simulink model "sampleModel653"  (R2023a)
settings: Solver=VariableStepAuto  StartTime=0.0  StopTime=10.0  RelTol=1e-3
undefined symbols (not defined in the file): DiscIntNeverNeededParam, magnitude, Newton, Raphson
libraries: simulink x238, slpidlib x68
(part 8 of 11)

== system sampleModel653/cfblk160/cfblk6 ==
  cfblk1 : Inport
  cfblk8 : Inport  Port=2
  cfblk3 : Delay  SampleTime=1
  cfblk4 : DiscreteFir  SampleTime=1
  cfblk5 : DiscreteFilter  SampleTime=1
  cfblk6 : Abs  SaturateOnIntegerOverflow=off
  cfblk7 : Signum
  cfblk2 : Outport
  cfblk9 : Outport  Port=2
  cfblk10 : Outport  Port=3
  wires:
  cfblk3/1 -> cfblk9/1
  cfblk1/1 -> cfblk6/1
  cfblk8/1 -> cfblk7/1, cfblk5/1
  cfblk5/1 -> cfblk2/1
  cfblk7/1 -> cfblk10/1
  cfblk6/1 -> cfblk4/1
  cfblk4/1 -> cfblk3/1

== system sampleModel653/cfblk160/cfblk7 ==
  cfblk1 : Inport
  cfblk7 : Inport  Port=2
  cfblk3 : slpidlib/PID Controller  Controller=PID  Form=Parallel  TimeDomain=Discrete-time  UseExternalTs=off  SampleTime=1  IntegratorMethod=Forward Euler  FilterMethod=Forward Euler  ControllerParametersSource=internal  P=1  I=1  UseKiTs=off  D=0  N=100  UseFilter=on  TunerSelectOption=Transfer Function Based (PID Tuner App)  InitialConditionSource=internal  InitialConditionForIntegrator=0  InitialConditionForFilter=0  DifferentiatorICPrevScaledInput=0  ExternalReset=none  TrackingMode=off  Kt=1  LimitOutput=off  SatLimitsSource=internal  UpperSaturationLimit=inf  LowerSaturationLimit=-inf  LinearizeAsGain=off  AntiWindupMode=none  Kb=1  LimitIntegrator=off  UpperIntegratorSaturationLimit=inf  LowerIntegratorSaturationLimit=-inf  POutMin=[]  POutMax=[]  IOutMin=[]  IOutMax=[]  DOutMin=[]  DOutMax=[]  NOutMin=[]  NOutMax=[]  SumOutMin=[]  SumOutMax=[]  SaturationOutMin=[]  SaturationOutMax=[]  PParamMin=[]  PParamMax=[]  IParamMin=[]  IParamMax=[]  DParamMin=[]  DParamMax=[]  NParamMin=[]  NParamMax=[]  KbParamMin=[]  KbParamMax=[]  KtParamMin=[]  KtParamMax=[]  KbOutMin=[]  KbOutMax=[]  KtOutMin=[]  KtOutMax=[]  IntegratorOutMin=[]  IntegratorOutMax=[]  FilterOutMin=[]  FilterOutMax=[]  SumI1OutMin=[]  SumI1OutMax=[]  SumI2OutMin=[]  SumI2OutMax=[]  SumI3OutMin=[]  SumI3OutMax=[]  SumI4OutMin=[]  SumI4OutMax=[]  SumDOutMin=[]  SumDOutMax=[]  DifferentiatorOutMin=[]  DifferentiatorOutMax=[]  FilterDiffOutCoefMin=[]  FilterDiffOutCoefMax=[]  ReciprocalOutMin=[]  ReciprocalOutMax=[]  SumDenOutMin=[]  SumDenOutMax=[]  SumNumOutMin=[]  SumNumOutMax=[]  DivideOutMin=[]  DivideOutMax=[]  UdiffTsProdOutMin=[]  UdiffTsProdOutMax=[]  NTsProdOutMin=[]  NTsProdOutMax=[]  UintegralTsProdOutMin=[]  UintegralTsProdOutMax=[]  UngainTsProdOutMin=[]  UngainTsProdOutMax=[]  ClampingZeroOutDataTypeStr=Inherit: Inherit via back propagation  ClampingZeroOutMin=[]  ClampingZeroOutMax=[]  FilterDenConstantOutDataTypeStr=Inherit: Inherit via back propagation  FilterDenConstantOutMin=[]  FilterDenConstantOutMax=[]  PCopyOutDataTypeStr=Inherit: Inherit via back propagation  PCopyOutMin=[]  PCopyOutMax=[]  NCopyOutDataTypeStr=Inherit: Inherit via back propagation  NCopyOutMin=[]  NCopyOutMax=[]  IntegratorContinuousStateAttributes=''  IntegratorStateMustResolveToSignalObject=off  IntegratorRTWStateStorageClass=Auto  FilterContinuousStateAttributes=''  FilterStateMustResolveToSignalObject=off  FilterRTWStateStorageClass=Auto  ParallelPVariant=InternalParameters  IdealPVariant=Disabled  IVariant=InternalParameters  DVariant=InternalParameters  IntegratorVariant=Discrete  SatVariant=Disabled  AWVariant=Passthrough  PCopyVariant=Disabled  TRVariant=Disabled  FdbkBlocksVariant=Forward  IdealPFdbkVariant=Disabled  SatFdbkVariant=Disabled  DerivativeFilterVariant=ForwardEulerFilter  NVariant=InternalParameters  NCopyVariant=Disabled  FilterICVariant=InternalICsFilter  IntegratorICVariant=InternalICs  ExternalResetVariant=Disabled  TRSumVariant=Passthrough  SumFdbkVariant=Disabled  SumVariant=Sum_PID  TsampFilterVariant=InternalTs  TsampNgainVariant=Passthrough  TsampIntegralVariant=Disabled_SignalSpec  ExternalSaturationOutDataTypeStr=Inherit: Same as second input
      settings: LibrarySourceBlock=simulink/Discrete/Discrete PID Controller
  cfblk4 : Sum  Inputs=|++
  cfblk5 : Polyval  Coefs=[ +2.081618890e-019, -1.441693666e-014, +4.719686976e-010, -8.536869453e-006, +1.621573104e-001, -8.087801117e+001 ]
  cfblk6 : Constant  Value=[-549633033.894766]  SampleTime=1
  cfblk2 : Outport
  wires:
  cfblk6/1 -> cfblk2/1
  cfblk7/1 -> cfblk3/1
  cfblk3/1 -> cfblk4/1
  cfblk1/1 -> cfblk4/2
  cfblk4/1 -> cfblk5/1

== system sampleModel653/cfblk161/cfblk13 ==
  cfblk1 : Inport
  cfblk13 : Inport  Port=2
  cfblk10 : Product
  cfblk11 : Constant  Value=[950367817.436596]  SampleTime=1
  cfblk12 : Constant  Value=[-836391739.954289]  SampleTime=1
  cfblk16 : Delay  SampleTime=1
  cfblk17 : Delay  SampleTime=1
  cfblk3 : PropagationDelay  SampleTime=1
  cfblk4 : simulink/Discrete/Transfer Fcn First Order  PoleZ=0.95  ICPrevOutput=0.0  DoSatur=off
  cfblk5 : simulink/Discrete/Tapped Delay  vinit=0.0  samptime=-1  NumDelays=1  DelayOrder=Oldest  includeCurrent=off
  cfblk6 : PropagationDelay  SampleTime=1
  cfblk7 : Sum  Inputs=+-
  cfblk8 : ComplexToMagnitudeAngle
  cfblk9 : Sqrt
  cfblk2 : Outport
  cfblk14 : Outport  Port=2
  cfblk15 : Outport  Port=3
  wires:
  cfblk3/1 -> cfblk4/1
  cfblk12/1 -> cfblk9/1
  cfblk1/1 -> cfblk6/1
  cfblk7/1 -> cfblk8/1
  cfblk13/1 -> cfblk15/1
  cfblk5/1 -> cfblk14/1, cfblk10/2
  cfblk4/1 -> cfblk6/2
  cfblk6/1 -> cfblk2/1
  cfblk8/2 -> cfblk10/1
  cfblk9/1 -> cfblk7/2, cfblk3/2
  cfblk11/1 -> cfblk3/1
  cfblk10/1 -> cfblk16/1
  cfblk16/1 -> cfblk5/1
  cfblk8/1 -> cfblk17/1
  cfblk17/1 -> cfblk7/1

== system sampleModel653/cfblk161/cfblk14 ==
  cfblk1 : Inport
  cfblk6 : Inport  Port=2
  cfblk3 : MinMax  Function=max  Inputs=3
  cfblk4 : Constant  Value=[-385450428.732004]  SampleTime=1
  cfblk5 : Constant  Value=[-397891502.363819]  SampleTime=1
  cfblk2 : Outport
  cfblk7 : Outport  Port=2
  cfblk8 : Outport  Port=3
  wires:
  cfblk5/1 -> cfblk7/1
  cfblk6/1 -> cfblk8/1, cfblk3/2
  cfblk1/1 -> cfblk2/1
  cfblk4/1 -> cfblk3/1, cfblk3/3

== system sampleModel653/cfblk162/cfblk10 ==
  cfblk1 : Inport
  cfblk6 : Inport  Port=2
  cfblk3 : DiscreteIntegrator  ICPrevOutput=DiscIntNeverNeededParam  ICPrevScaledInput=DiscIntNeverNeededParam
  cfblk4 : Sqrt  Operator=rSqrt  AlgorithmType=Newton-Raphson
  cfblk5 : Sum  Inputs=--
  cfblk2 : Outport
  cfblk7 : Outport  Port=2
  wires:
  cfblk1/1 -> cfblk4/1
  cfblk6/1 -> cfblk2/1, cfblk5/2
  cfblk3/1 -> cfblk7/1, cfblk5/1
  cfblk4/1 -> cfblk3/1

== system sampleModel653/cfblk162/cfblk11 ==
  cfblk1 : Inport
  cfblk14 : Inport  Port=2
  cfblk15 : Inport  Port=3
  cfblk16 : Inport  Port=4
  cfblk10 : Gain  Gain=[646766458.075510]
  cfblk11 : Constant  Value=[-624023355.603475]  SampleTime=1
  cfblk12 : Constant  Value=[-240685083.837348]  SampleTime=1
  cfblk13 : Constant  Value=[301386795.855852]  SampleTime=1
  cfblk3 : DiscreteIntegrator  ICPrevOutput=DiscIntNeverNeededParam  ICPrevScaledInput=DiscIntNeverNeededParam
  cfblk4 : UnaryMinus
  cfblk5 : Trigonometry
  cfblk6 : Math  Operator=rem
  cfblk7 : UnaryMinus
  cfblk8 : Signum
  cfblk9 : simulink/Math Operations/Slider Gain  gain=1  low=0  high=2
  cfblk2 : Outport
  wires:
  cfblk15/1 -> cfblk6/1
  cfblk12/1 -> cfblk6/2
  cfblk16/1 -> cfblk2/1
  cfblk4/1 -> cfblk9/1
  cfblk14/1 -> cfblk7/1
  cfblk10/1 -> cfblk3/1
  cfblk11/1 -> cfblk4/1
  cfblk13/1 -> cfblk10/1
  cfblk6/1 -> cfblk8/1
  cfblk9/1 -> cfblk5/1

== system sampleModel653/cfblk162/cfblk7 ==
  cfblk1 : Inport
  cfblk13 : Inport  Port=2
  cfblk14 : Inport  Port=3
  cfblk10 : PermuteDimensions
  cfblk11 : Constant  Value=[11170143.397461]  SampleTime=1
  cfblk12 : Constant  Value=[-707565245.150474]  SampleTime=1
  cfblk17 : Delay  SampleTime=1
  cfblk3 : DiscreteTransferFcn  SampleTime=1
  cfblk4 : ComplexToMagnitudeAngle
  cfblk5 : DotProduct  OutDataTypeStr=Inherit: Inherit via internal rule
  cfblk6 : Bias  Bias=[-243802448.870084]  SaturateOnIntegerOverflow=off
  cfblk7 : Bias  Bias=[722005986.652119]  SaturateOnIntegerOverflow=off
  cfblk8 : Sum  Inputs=+-
  cfblk9 : PermuteDimensions
  cfblk2 : Outport
  cfblk15 : Outport  Port=2
  cfblk16 : Outport  Port=3
  wires:
  cfblk3/1 -> cfblk10/1
  cfblk1/1 -> cfblk3/1
  cfblk10/1 -> cfblk5/2
  cfblk13/1 -> cfblk6/1
  cfblk7/1 -> cfblk15/1
  cfblk14/1 -> cfblk2/1
  cfblk4/1 -> cfblk9/1
  cfblk11/1 -> cfblk16/1
  cfblk6/1 -> cfblk4/1
  cfblk12/1 -> cfblk7/1
  cfblk4/2 -> cfblk8/1
  cfblk5/1 -> cfblk8/2
  cfblk8/1 -> cfblk17/1
  cfblk17/1 -> cfblk5/1

== system sampleModel653/cfblk162/cfblk8 ==
  cfblk1 : Inport
  cfblk7 : Inport  Port=2
  cfblk8 : Inport  Port=3
  cfblk3 : DiscreteFilter  SampleTime=1
  cfblk4 : PermuteDimensions
  cfblk5 : Trigonometry
  cfblk6 : Constant  Value=[643614640.202509]  SampleTime=1
  cfblk2 : Outport
  cfblk9 : Outport  Port=2
  cfblk10 : Outport  Port=3
  wires:
  cfblk8/1 -> cfblk3/1
  cfblk3/1 -> cfblk2/1
  cfblk6/1 -> cfblk5/1
  cfblk7/1 -> cfblk9/1
  cfblk1/1 -> cfblk4/1
  cfblk5/1 -> cfblk10/1

== system sampleModel653/cfblk162/cfblk9 ==
  cfblk1 : Inport
  cfblk14 : Inport  Port=2
  cfblk15 : Inport  Port=3
  cfblk10 : Sum  Inputs=|++
  cfblk11 : Bias  Bias=[360480806.140065]  SaturateOnIntegerOverflow=off
  cfblk12 : Bias  Bias=[-571993292.003574]  SaturateOnIntegerOverflow=off
  cfblk13 : Constant  Value=[994996432.571754]  SampleTime=1
  cfblk18 : Delay  SampleTime=1
  cfblk3 : DiscreteStateSpace
  cfblk4 : DiscreteTransferFcn  SampleTime=1
  cfblk5 : Sum  Inputs=+-
  cfblk6 : PermuteDimensions
  cfblk7 : Product  Inputs=**
  cfblk8 : Polyval  Coefs=[ +2.081618890e-019, -1.441693666e-014, +4.719686976e-010, -8.536869453e-006, +1.621573104e-001, -8.087801117e+001 ]
  cfblk9 : simulink/Math Operations/Slider Gain  gain=1  low=0  high=2
  cfblk2 : Outport
  cfblk16 : Outport  Port=2
  cfblk17 : Outport  Port=3
  wires:
  cfblk7/1 -> cfblk9/1
  cfblk13/1 -> cfblk4/1
  cfblk15/1 -> cfblk16/1, cfblk5/2
  cfblk5/1 -> cfblk11/1
  cfblk14/1 -> cfblk17/1
  cfblk3/1 -> cfblk12/1, cfblk10/2
  cfblk11/1 -> cfblk6/1
  cfblk6/1 -> cfblk8/1
  cfblk8/1 -> cfblk7/2
  cfblk4/1 -> cfblk3/1
  cfblk9/1 -> cfblk10/1
  cfblk12/1 -> cfblk2/1
  cfblk1/1 -> cfblk5/1
  cfblk10/1 -> cfblk18/1
  cfblk18/1 -> cfblk7/1

== system sampleModel653/cfblk164/cfblk6 ==
  cfblk1 : Inport
  cfblk12 : Inport  Port=2
  cfblk13 : Inport  Port=3
  cfblk14 : Inport  Port=4
  cfblk15 : Inport  Port=5
  cfblk10 : Sum  Inputs=|++
  cfblk11 : Constant  Value=[-495831747.565326]  SampleTime=1
  cfblk16 : Delay  SampleTime=1
  cfblk3 : DiscreteZeroPole  Poles=[0 0.5]  Gain=1
  cfblk4 : Polyval  Coefs=[ +2.081618890e-019, -1.441693666e-014, +4.719686976e-010, -8.536869453e-006, +1.621573104e-001, -8.087801117e+001 ]
  cfblk5 : Product  Inputs=*
  cfblk6 : Polyval  Coefs=[ +2.081618890e-019, -1.441693666e-014, +4.719686976e-010, -8.536869453e-006, +1.621573104e-001, -8.087801117e+001 ]
  cfblk7 : MinMax
  cfblk8 : Sum  Inputs=+-
  cfblk9 : Gain  Gain=[160082621.041348]
  cfblk2 : Outport
  wires:
  cfblk12/1 -> cfblk6/1
  cfblk13/1 -> cfblk4/1
  cfblk4/1 -> cfblk2/1
  cfblk11/1 -> cfblk7/1
  cfblk15/1 -> cfblk9/1
  cfblk6/1 -> cfblk5/1
  cfblk3/1 -> cfblk8/1
  cfblk10/1 -> cfblk8/2
  cfblk9/1 -> cfblk10/1
  cfblk7/1 -> cfblk10/2
  cfblk8/1 -> cfblk16/1
  cfblk16/1 -> cfblk3/1

== system sampleModel653/cfblk165/cfblk7 ==
  cfblk1 : Inport
  cfblk3 : DiscreteTransferFcn  SampleTime=1
  cfblk4 : Gain  Gain=[-702568927.558802]
  cfblk5 : Product  Inputs=*
  cfblk8 : Delay  SampleTime=1
  cfblk2 : Outport
  cfblk6 : Outport  Port=2
  cfblk7 : Outport  Port=3
  wires:
  cfblk1/1 -> cfblk2/1, cfblk4/1
  cfblk4/1 -> cfblk7/1
  cfblk3/1 -> cfblk6/1, cfblk5/1
  cfblk5/1 -> cfblk8/1
  cfblk8/1 -> cfblk3/1

== system sampleModel653/cfblk166/cfblk7 ==
  cfblk1 : Inport
  cfblk10 : Inport  Port=2
  cfblk11 : Inport  Port=3
  cfblk12 : Inport  Port=4
  cfblk13 : Inport  Port=5
  cfblk14 : Inport  Port=6
  cfblk15 : Inport  Port=7
  cfblk3 : PropagationDelay  SampleTime=1
  cfblk4 : DiscreteFilter  SampleTime=1
  cfblk5 : DiscreteFilter  SampleTime=1
  cfblk6 : UnitDelay  HasFrameUpgradeWarning=on
  cfblk7 : PermuteDimensions
  cfblk8 : Bias  Bias=[88992789.129511]  SaturateOnIntegerOverflow=off
  cfblk9 : Constant  Value=[-39645168.443005]  SampleTime=1
  cfblk2 : Outport
  wires:
  cfblk12/1 -> cfblk8/1
  cfblk1/1 -> cfblk5/1
  cfblk10/1 -> cfblk6/1
  cfblk14/1 -> cfblk4/1
  cfblk11/1 -> cfblk3/1
  cfblk9/1 -> cfblk3/2
  cfblk4/1 -> cfblk7/1
  cfblk6/1 -> cfblk2/1

== system sampleModel653/cfblk167/cfblk10 ==
  cfblk1 : Inport
  cfblk9 : Inport  Port=2
  cfblk11 : Delay  SampleTime=1
  cfblk12 : Delay  SampleTime=1
  cfblk3 : PropagationDelay  SampleTime=1
  cfblk4 : PropagationDelay  SampleTime=1
  cfblk5 : DiscreteZeroPole  Poles=[0 0.5]  Gain=1
  cfblk6 : Product  Inputs=**
  cfblk7 : MinMax  Inputs=3
  cfblk8 : Sum  Inputs=|++
  cfblk2 : Outport
  cfblk10 : Outport  Port=2
  wires:
  cfblk9/1 -> cfblk5/1
  cfblk5/1 -> cfblk10/1
  cfblk3/1 -> cfblk4/1, cfblk8/1
  cfblk8/1 -> cfblk6/2, cfblk12/1
  cfblk4/1 -> cfblk6/1
  cfblk1/1 -> cfblk7/2, cfblk7/3
  cfblk7/1 -> cfblk2/1, cfblk3/1, cfblk3/2, cfblk8/2
  cfblk6/1 -> cfblk11/1
  cfblk11/1 -> cfblk4/2
  cfblk12/1 -> cfblk7/1

== system sampleModel653/cfblk167/cfblk11 ==
  cfblk1 : Inport
  cfblk14 : Inport  Port=2
  cfblk15 : Inport  Port=3
  cfblk10 : DotProduct  OutDataTypeStr=Inherit: Inherit via internal rule
  cfblk11 : Sqrt  Operator=rSqrt  AlgorithmType=Newton-Raphson
  cfblk12 : Sum  Inputs=|++
  cfblk13 : Product  Inputs=*
  cfblk{17..20} (4 alike) : Delay  SampleTime=1
  cfblk3 : DiscreteFilter  SampleTime=1
  cfblk4 : PropagationDelay  SampleTime=1
  cfblk5 : PropagationDelay  SampleTime=1
  cfblk6 : Signum
  cfblk7 : MinMax  Function=max  Inputs=2
  cfblk8 : Sum  Inputs=|++
  cfblk9 : DotProduct  OutDataTypeStr=Inherit: Inherit via internal rule
  cfblk2 : Outport
  cfblk16 : Outport  Port=2
  wires:
  cfblk9/1 -> cfblk8/1, cfblk7/1
  cfblk13/1 -> cfblk5/1, cfblk8/2, cfblk2/1
  cfblk8/1 -> cfblk7/2, cfblk18/1
  cfblk6/1 -> cfblk4/2
  cfblk4/1 -> cfblk10/1
  cfblk14/1 -> cfblk13/1
  cfblk1/1 -> cfblk3/1
  cfblk10/1 -> cfblk12/2, cfblk9/2
  cfblk3/1 -> cfblk16/1
  cfblk5/1 -> cfblk11/1
  cfblk12/1 -> cfblk9/1, cfblk17/1
  cfblk15/1 -> cfblk6/1
  cfblk17/1 -> cfblk10/2
  cfblk18/1 -> cfblk4/1
  cfblk7/1 -> cfblk19/1
  cfblk19/1 -> cfblk12/1
  cfblk11/1 -> cfblk20/1
  cfblk20/1 -> cfblk5/2

== system sampleModel653/cfblk167/cfblk12 ==
  cfblk1 : Inport
  cfblk10 : Inport  Port=2
  cfblk11 : Inport  Port=3
  cfblk12 : Delay  SampleTime=1
  cfblk3 : Product
  cfblk4 : simulink/Math Operations/MinMax Running Resettable  Function=min  vinit=0.0
  cfblk5 : Assignment  DiagnosticForDimensions=Warning  IndexOptions=Index vector (dialog)  Indices=1  OutputSizes=1
  cfblk6 : Math  Operator=hermitian
  cfblk7 : MinMax  Inputs=2
  cfblk8 : Constant  Value=[598638791.234022]  SampleTime=1
  cfblk9 : Constant  Value=[471752082.064048]  SampleTime=1
  cfblk2 : Outport
  wires:
  cfblk8/1 -> cfblk7/1
  cfblk9/1 -> cfblk6/1
  cfblk1/1 -> cfblk7/2
  cfblk3/1 -> cfblk5/1
  cfblk6/1 -> cfblk3/1
  cfblk10/1 -> cfblk5/2
  cfblk11/1 -> cfblk4/1
  cfblk5/1 -> cfblk4/2
  cfblk7/1 -> cfblk2/1
  cfblk4/1 -> cfblk12/1
  cfblk12/1 -> cfblk3/2

== system sampleModel653/cfblk167/cfblk13 ==
  cfblk1 : Inport
  cfblk15 : Inport  Port=2
  cfblk16 : Inport  Port=3
  cfblk10 : Trigonometry
  cfblk11 : MinMax  Function=max  Inputs=2
  cfblk12 : Assignment  DiagnosticForDimensions=Warning  IndexOptions=Index vector (dialog)  Indices=1  OutputSizes=1
  cfblk13 : Constant  Value=[580497405.905219]  SampleTime=1
  cfblk14 : Constant  Value=[-757720306.002820]  SampleTime=1
  cfblk3 : UnitDelay  HasFrameUpgradeWarning=on
  cfblk4 : Gain  Gain=[619591310.488416]
  cfblk5 : DotProduct  OutDataTypeStr=Inherit: Inherit via internal rule
  cfblk6 : Math  Operator=10^u
  cfblk7 : PermuteDimensions
  cfblk8 : Product  Inputs=*
  cfblk9 : Sqrt  Operator=rSqrt  AlgorithmType=Newton-Raphson
  cfblk2 : Outport
  cfblk17 : Outport  Port=2
  wires:
  cfblk6/1 -> cfblk8/1
  cfblk14/1 -> cfblk12/1
  cfblk4/1 -> cfblk10/1
  cfblk10/1 -> cfblk7/1
  cfblk9/1 -> cfblk12/2
  cfblk15/1 -> cfblk9/1
  cfblk1/1 -> cfblk5/1
  cfblk11/1 -> cfblk6/1
  cfblk5/1 -> cfblk4/1
  cfblk8/1 -> cfblk17/1
  cfblk7/1 -> cfblk3/1
  cfblk13/1 -> cfblk2/1
  cfblk3/1 -> cfblk11/1
  cfblk16/1 -> cfblk11/2
  cfblk12/1 -> cfblk5/2

== system sampleModel653/cfblk167/cfblk18 ==
  cfblk1 : Inport
  cfblk10 : Inport  Port=2
  cfblk11 : Inport  Port=3
  cfblk12 : Inport  Port=4
  Action Port : ActionPort  ActionPortLabel=if(u1 >= 0)
  cfblk3 : simulink/Discrete/Transfer Fcn First Order  PoleZ=0.95  ICPrevOutput=0.0  DoSatur=off
  cfblk4 : DiscreteFir
  cfblk5 : Delay  ShowEnablePort=on
      settings: InputPortMap=u0,e6
  cfblk6 : DiscreteZeroPole  Poles=[0 0.5]  Gain=1  SampleTime=-1
  cfblk7 : Polyval  Coefs=[ +2.081618890e-019, -1.441693666e-014, +4.719686976e-010, -8.536869453e-006, +1.621573104e-001, -8.087801117e+001 ]
  cfblk8 : Constant  Value=[815668544.395762]  SampleTime=1
  cfblk9 : Constant  Value=[749946664.486062]  SampleTime=1
  cfblk2 : Outport
  cfblk13 : Outport  Port=2
  wires:
  cfblk10/1 -> cfblk5/1
  cfblk4/1 -> cfblk13/1
  cfblk12/1 -> cfblk5/2
  cfblk8/1 -> cfblk6/1
  cfblk11/1 -> cfblk7/1
  cfblk5/1 -> cfblk4/1
  cfblk3/1 -> cfblk2/1
  cfblk6/1 -> cfblk3/1

== system sampleModel653/cfblk167/cfblk19 ==
  cfblk1 : Inport
  cfblk13 : Inport  Port=2
  cfblk14 : Inport  Port=3
  cfblk15 : Inport  Port=4
  Action Port : ActionPort  ActionPortLabel=else
  cfblk10 : Product
  cfblk11 : Constant  Value=[365730879.526834]  SampleTime=1
  cfblk12 : Constant  Value=[357784295.505413]  SampleTime=1
  cfblk18 : Delay
  cfblk3 : PropagationDelay  SampleTime=-1
  cfblk4 : slpidlib/PID Controller  Controller=PID  Form=Parallel  TimeDomain=Discrete-time  UseExternalTs=off  SampleTime=-1  IntegratorMethod=Forward Euler  FilterMethod=Forward Euler  ControllerParametersSource=internal  P=1  I=1  UseKiTs=off  D=0  N=100  UseFilter=on  TunerSelectOption=Transfer Function Based (PID Tuner App)  InitialConditionSource=internal  InitialConditionForIntegrator=0  InitialConditionForFilter=0  DifferentiatorICPrevScaledInput=0  ExternalReset=none  TrackingMode=off  Kt=1  LimitOutput=off  SatLimitsSource=internal  UpperSaturationLimit=inf  LowerSaturationLimit=-inf  LinearizeAsGain=off  AntiWindupMode=none  Kb=1  LimitIntegrator=off  UpperIntegratorSaturationLimit=inf  LowerIntegratorSaturationLimit=-inf  POutMin=[]  POutMax=[]  IOutMin=[]  IOutMax=[]  DOutMin=[]  DOutMax=[]  NOutMin=[]  NOutMax=[]  SumOutMin=[]  SumOutMax=[]  SaturationOutMin=[]  SaturationOutMax=[]  PParamMin=[]  PParamMax=[]  IParamMin=[]  IParamMax=[]  DParamMin=[]  DParamMax=[]  NParamMin=[]  NParamMax=[]  KbParamMin=[]  KbParamMax=[]  KtParamMin=[]  KtParamMax=[]  KbOutMin=[]  KbOutMax=[]  KtOutMin=[]  KtOutMax=[]  IntegratorOutMin=[]  IntegratorOutMax=[]  FilterOutMin=[]  FilterOutMax=[]  SumI1OutMin=[]  SumI1OutMax=[]  SumI2OutMin=[]  SumI2OutMax=[]  SumI3OutMin=[]  SumI3OutMax=[]  SumI4OutMin=[]  SumI4OutMax=[]  SumDOutMin=[]  SumDOutMax=[]  DifferentiatorOutMin=[]  DifferentiatorOutMax=[]  FilterDiffOutCoefMin=[]  FilterDiffOutCoefMax=[]  ReciprocalOutMin=[]  ReciprocalOutMax=[]  SumDenOutMin=[]  SumDenOutMax=[]  SumNumOutMin=[]  SumNumOutMax=[]  DivideOutMin=[]  DivideOutMax=[]  UdiffTsProdOutMin=[]  UdiffTsProdOutMax=[]  NTsProdOutMin=[]  NTsProdOutMax=[]  UintegralTsProdOutMin=[]  UintegralTsProdOutMax=[]  UngainTsProdOutMin=[]  UngainTsProdOutMax=[]  ClampingZeroOutDataTypeStr=Inherit: Inherit via back propagation  ClampingZeroOutMin=[]  ClampingZeroOutMax=[]  FilterDenConstantOutDataTypeStr=Inherit: Inherit via back propagation  FilterDenConstantOutMin=[]  FilterDenConstantOutMax=[]  PCopyOutDataTypeStr=Inherit: Inherit via back propagation  PCopyOutMin=[]  PCopyOutMax=[]  NCopyOutDataTypeStr=Inherit: Inherit via back propagation  NCopyOutMin=[]  NCopyOutMax=[]  IntegratorContinuousStateAttributes=''  IntegratorStateMustResolveToSignalObject=off  IntegratorRTWStateStorageClass=Auto  FilterContinuousStateAttributes=''  FilterStateMustResolveToSignalObject=off  FilterRTWStateStorageClass=Auto  ParallelPVariant=InternalParameters  IdealPVariant=Disabled  IVariant=InternalParameters  DVariant=InternalParameters  IntegratorVariant=Discrete  SatVariant=Disabled  AWVariant=Passthrough  PCopyVariant=Disabled  TRVariant=Disabled  FdbkBlocksVariant=Forward  IdealPFdbkVariant=Disabled  SatFdbkVariant=Disabled  DerivativeFilterVariant=ForwardEulerFilter  NVariant=InternalParameters  NCopyVariant=Disabled  FilterICVariant=InternalICsFilter  IntegratorICVariant=InternalICs  ExternalResetVariant=Disabled  TRSumVariant=Passthrough  SumFdbkVariant=Disabled  SumVariant=Sum_PID  TsampFilterVariant=InternalTs  TsampNgainVariant=Passthrough  TsampIntegralVariant=Disabled_SignalSpec  ExternalSaturationOutDataTypeStr=Inherit: Same as second input
      settings: LibrarySourceBlock=simulink/Discrete/Discrete PID Controller
  cfblk5 : Delay
  cfblk6 : DiscreteStateSpace  SampleTime=-1
  cfblk7 : UnitDelay  SampleTime=-1  HasFrameUpgradeWarning=on
  cfblk8 : Signum
  cfblk9 : Sum  Inputs=+
  cfblk2 : Outport
  cfblk16 : Outport  Port=2
  cfblk17 : Outport  Port=3
  wires:
  cfblk9/1 -> cfblk10/1
  cfblk12/1 -> cfblk5/1
  cfblk5/1 -> cfblk10/2
  cfblk13/1 -> cfblk4/1
  cfblk11/1 -> cfblk17/1
  cfblk1/1 -> cfblk16/1
  cfblk14/1 -> cfblk7/1
  cfblk6/1 -> cfblk2/1
  cfblk7/1 -> cfblk6/1
  cfblk8/1 -> cfblk3/1
  cfblk3/1 -> cfblk9/1
  cfblk15/1 -> cfblk8/1
  cfblk10/1 -> cfblk18/1
  cfblk18/1 -> cfblk3/2

== system sampleModel653/cfblk167/cfblk8 ==
  cfblk1 : Inport
  cfblk3 : DiscreteFir  SampleTime=1
  cfblk4 : simulink/Discrete/Tapped Delay  vinit=0.0  samptime=-1  NumDelays=1  DelayOrder=Oldest  includeCurrent=off
  cfblk5 : Sqrt
  cfblk6 : Rounding
  cfblk9 : Delay  SampleTime=1
  cfblk2 : Outport
  cfblk7 : Outport  Port=2
  cfblk8 : Outport  Port=3
  wires:
  cfblk6/1 -> cfblk5/1, cfblk9/1
  cfblk3/1 -> cfblk6/1
  cfblk5/1 -> cfblk2/1
  cfblk1/1 -> cfblk4/1
  cfblk4/1 -> cfblk8/1, cfblk7/1
  cfblk9/1 -> cfblk3/1

== system sampleModel653/cfblk167/cfblk9 ==
  cfblk1 : Inport
  cfblk11 : Inport  Port=2
  cfblk12 : Inport  Port=3
  cfblk13 : Inport  Port=4
  cfblk14 : Inport  Port=5
  cfblk10 : Constant  Value=[484188899.570974]  SampleTime=1
  cfblk3 : Sin  TimeSource=Use external signal  SampleTime=0
  cfblk4 : Squeeze
  cfblk5 : Squeeze
  cfblk6 : Sum  Inputs=|++
  cfblk7 : Polyval  Coefs=[ +2.081618890e-019, -1.441693666e-014, +4.719686976e-010, -8.536869453e-006, +1.621573104e-001, -8.087801117e+001 ]
  cfblk8 : Sqrt  Operator=rSqrt  AlgorithmType=Newton-Raphson
  cfblk9 : Constant  Value=[327374608.869159]  SampleTime=1
  cfblk2 : Outport
  cfblk15 : Outport  Port=2
  wires:
  cfblk9/1 -> cfblk2/1
  cfblk4/1 -> cfblk8/1
  cfblk5/1 -> cfblk4/1
  cfblk10/1 -> cfblk6/1
  cfblk7/1 -> cfblk15/1
  cfblk12/1 -> cfblk3/1
  cfblk11/1 -> cfblk5/1
  cfblk6/1 -> cfblk7/1
  cfblk3/1 -> cfblk6/2

== system sampleModel653/cfblk168/cfblk7 ==
  cfblk1 : Inport
  cfblk10 : Constant  Value=[701061649.043973]  SampleTime=1
  cfblk12 : Delay  SampleTime=1
  cfblk13 : Delay  SampleTime=1
  cfblk3 : slpidlib/PID Controller  Controller=PID  Form=Parallel  TimeDomain=Discrete-time  UseExternalTs=off  SampleTime=1  IntegratorMethod=Forward Euler  FilterMethod=Forward Euler  ControllerParametersSource=internal  P=1  I=1  UseKiTs=off  D=0  N=100  UseFilter=on  TunerSelectOption=Transfer Function Based (PID Tuner App)  InitialConditionSource=internal  InitialConditionForIntegrator=0  InitialConditionForFilter=0  DifferentiatorICPrevScaledInput=0  ExternalReset=none  TrackingMode=off  Kt=1  LimitOutput=off  SatLimitsSource=internal  UpperSaturationLimit=inf  LowerSaturationLimit=-inf  LinearizeAsGain=off  AntiWindupMode=none  Kb=1  LimitIntegrator=off  UpperIntegratorSaturationLimit=inf  LowerIntegratorSaturationLimit=-inf  POutMin=[]  POutMax=[]  IOutMin=[]  IOutMax=[]  DOutMin=[]  DOutMax=[]  NOutMin=[]  NOutMax=[]  SumOutMin=[]  SumOutMax=[]  SaturationOutMin=[]  SaturationOutMax=[]  PParamMin=[]  PParamMax=[]  IParamMin=[]  IParamMax=[]  DParamMin=[]  DParamMax=[]  NParamMin=[]  NParamMax=[]  KbParamMin=[]  KbParamMax=[]  KtParamMin=[]  KtParamMax=[]  KbOutMin=[]  KbOutMax=[]  KtOutMin=[]  KtOutMax=[]  IntegratorOutMin=[]  IntegratorOutMax=[]  FilterOutMin=[]  FilterOutMax=[]  SumI1OutMin=[]  SumI1OutMax=[]  SumI2OutMin=[]  SumI2OutMax=[]  SumI3OutMin=[]  SumI3OutMax=[]  SumI4OutMin=[]  SumI4OutMax=[]  SumDOutMin=[]  SumDOutMax=[]  DifferentiatorOutMin=[]  DifferentiatorOutMax=[]  FilterDiffOutCoefMin=[]  FilterDiffOutCoefMax=[]  ReciprocalOutMin=[]  ReciprocalOutMax=[]  SumDenOutMin=[]  SumDenOutMax=[]  SumNumOutMin=[]  SumNumOutMax=[]  DivideOutMin=[]  DivideOutMax=[]  UdiffTsProdOutMin=[]  UdiffTsProdOutMax=[]  NTsProdOutMin=[]  NTsProdOutMax=[]  UintegralTsProdOutMin=[]  UintegralTsProdOutMax=[]  UngainTsProdOutMin=[]  UngainTsProdOutMax=[]  ClampingZeroOutDataTypeStr=Inherit: Inherit via back propagation  ClampingZeroOutMin=[]  ClampingZeroOutMax=[]  FilterDenConstantOutDataTypeStr=Inherit: Inherit via back propagation  FilterDenConstantOutMin=[]  FilterDenConstantOutMax=[]  PCopyOutDataTypeStr=Inherit: Inherit via back propagation  PCopyOutMin=[]  PCopyOutMax=[]  NCopyOutDataTypeStr=Inherit: Inherit via back propagation  NCopyOutMin=[]  NCopyOutMax=[]  IntegratorContinuousStateAttributes=''  IntegratorStateMustResolveToSignalObject=off  IntegratorRTWStateStorageClass=Auto  FilterContinuousStateAttributes=''  FilterStateMustResolveToSignalObject=off  FilterRTWStateStorageClass=Auto  ParallelPVariant=InternalParameters  IdealPVariant=Disabled  IVariant=InternalParameters  DVariant=InternalParameters  IntegratorVariant=Discrete  SatVariant=Disabled  AWVariant=Passthrough  PCopyVariant=Disabled  TRVariant=Disabled  FdbkBlocksVariant=Forward  IdealPFdbkVariant=Disabled  SatFdbkVariant=Disabled  DerivativeFilterVariant=ForwardEulerFilter  NVariant=InternalParameters  NCopyVariant=Disabled  FilterICVariant=InternalICsFilter  IntegratorICVariant=InternalICs  ExternalResetVariant=Disabled  TRSumVariant=Passthrough  SumFdbkVariant=Disabled  SumVariant=Sum_PID  TsampFilterVariant=InternalTs  TsampNgainVariant=Passthrough  TsampIntegralVariant=Disabled_SignalSpec  ExternalSaturationOutDataTypeStr=Inherit: Same as second input
      settings: LibrarySourceBlock=simulink/Discrete/Discrete PID Controller
  cfblk4 : Delay  DelayLengthSource=Input port  SampleTime=1
      settings: InputPortMap=u0,p1
  cfblk5 : DiscreteFir  SampleTime=1
  cfblk6 : Assignment  DiagnosticForDimensions=Warning  IndexOptions=Index vector (dialog)  Indices=1  OutputSizes=1
  cfblk7 : UnaryMinus
  cfblk8 : Reshape
  cfblk9 : Rounding
  cfblk2 : Outport
  cfblk11 : Outport  Port=2
  wires:
  cfblk4/1 -> cfblk6/1
  cfblk3/1 -> cfblk5/1
  cfblk1/1 -> cfblk6/2
  cfblk7/1 -> cfblk9/1
  cfblk6/1 -> cfblk2/1
  cfblk9/1 -> cfblk4/1, cfblk8/1
  cfblk8/1 -> cfblk11/1, cfblk13/1
  cfblk10/1 -> cfblk4/2
  cfblk5/1 -> cfblk12/1
  cfblk12/1 -> cfblk3/1
  cfblk13/1 -> cfblk7/1

== system sampleModel653/cfblk168/cfblk8 ==
  cfblk1 : Inport
  cfblk10 : Inport  Port=2
  cfblk12 : Delay  SampleTime=1
  cfblk3 : DiscreteIntegrator  ICPrevOutput=DiscIntNeverNeededParam  ICPrevScaledInput=DiscIntNeverNeededParam
  cfblk4 : simulink/Discrete/Transfer Fcn First Order  PoleZ=0.95  ICPrevOutput=0.0  DoSatur=off
  cfblk5 : Delay  DelayLengthSource=Input port  SampleTime=1
      settings: InputPortMap=u0,p1
  cfblk6 : Bias  Bias=[-161283541.560925]  SaturateOnIntegerOverflow=off
  cfblk7 : Product
  cfblk8 : ComplexToMagnitudeAngle
  cfblk9 : Constant  Value=[-84826546.757724]  SampleTime=1
  cfblk2 : Outport
  cfblk11 : Outport  Port=2
  wires:
  cfblk8/1 -> cfblk11/1
  cfblk3/1 -> cfblk4/1
  cfblk8/2 -> cfblk2/1
  cfblk10/1 -> cfblk5/1
  cfblk5/1 -> cfblk6/1
  cfblk4/1 -> cfblk8/1
  cfblk7/1 -> cfblk3/1
  cfblk9/1 -> cfblk7/1
  cfblk1/1 -> cfblk7/2
  cfblk6/1 -> cfblk12/1
  cfblk12/1 -> cfblk5/2

== system sampleModel653/cfblk168/cfblk9 ==
  cfblk1 : Inport
  cfblk8 : Inport  Port=2
  cfblk10 : Delay  SampleTime=1
  cfblk3 : Delay  SampleTime=1
  cfblk4 : Sqrt  Operator=rSqrt  AlgorithmType=Newton-Raphson
  cfblk5 : simulink/Math Operations/MinMax Running Resettable  Function=min  vinit=0.0
  cfblk6 : simulink/Math Operations/Slider Gain  gain=1  low=0  high=2
  cfblk7 : Constant  Value=[295495692.389129]  SampleTime=1
  cfblk2 : Outport
  cfblk9 : Outport  Port=2
  wires:
  cfblk8/1 -> cfblk9/1
  cfblk1/1 -> cfblk5/1
  cfblk3/1 -> cfblk4/1
  cfblk7/1 -> cfblk5/2
  cfblk4/1 -> cfblk6/1
  cfblk5/1 -> cfblk2/1
  cfblk6/1 -> cfblk10/1
  cfblk10/1 -> cfblk3/1

== system sampleModel653/cfblk169/cfblk5 ==
  cfblk1 : Inport
  cfblk10 : Delay  SampleTime=1
  cfblk11 : Delay  SampleTime=1
  cfblk3 : PropagationDelay  SampleTime=1
  cfblk4 : simulink/Discrete/Transfer Fcn Lead or Lag  PoleZ=0.95  ZeroZ=0.75  ICPrevOutput=0.0  ICPrevInput=0.0  DoSatur=off
  cfblk5 : Sqrt  Operator=rSqrt  AlgorithmType=Newton-Raphson
  cfblk6 : Abs  SaturateOnIntegerOverflow=off
  cfblk7 : Squeeze
  cfblk8 : Sum  Inputs=-+
  cfblk9 : Product  Inputs=**
  cfblk2 : Outport
  wires:
  cfblk6/1 -> cfblk2/1
  cfblk7/1 -> cfblk4/1, cfblk11/1
  cfblk8/1 -> cfblk6/1, cfblk3/1
  cfblk5/1 -> cfblk7/1
  cfblk1/1 -> cfblk8/2, cfblk3/2
  cfblk3/1 -> cfblk9/1
  cfblk4/1 -> cfblk9/2
  cfblk9/1 -> cfblk10/1
  cfblk10/1 -> cfblk8/1
  cfblk11/1 -> cfblk5/1

== system sampleModel653/cfblk169/cfblk6 ==
  cfblk1 : Inport
  cfblk9 : Inport  Port=2
  cfblk10 : Inport  Port=3
  cfblk3 : Delay  SampleTime=1
  cfblk4 : ComplexToMagnitudeAngle
  cfblk5 : Constant  Value=[397897555.696305]  SampleTime=1
  cfblk6 : Constant  Value=[772429863.008263]  SampleTime=1
  cfblk7 : Constant  Value=[-755008844.378157]  SampleTime=1
  cfblk8 : Constant  Value=[-741770211.228956]  SampleTime=1
  cfblk2 : Outport
  cfblk11 : Outport  Port=2
  cfblk12 : Outport  Port=3
  cfblk13 : Outport  Port=4
  wires:
  cfblk9/1 -> cfblk11/1
  cfblk8/1 -> cfblk12/1
  cfblk4/1 -> cfblk2/1
  cfblk10/1 -> cfblk3/1
  cfblk1/1 -> cfblk4/1
  cfblk7/1 -> cfblk13/1

== system sampleModel653/cfblk170/cfblk10 ==
  cfblk1 : Inport
  cfblk13 : Inport  Port=2
  cfblk14 : Inport  Port=3
  cfblk15 : Inport  Port=4
  cfblk10 : simulink/Math Operations/Slider Gain  gain=1  low=0  high=2
  cfblk11 : PermuteDimensions
  cfblk12 : Constant  Value=[-575625179.417176]  SampleTime=1
  cfblk3 : DiscreteZeroPole  Poles=[0 0.5]  Gain=1
  cfblk4 : Delay  DelayLengthSource=Input port  SampleTime=1
      settings: InputPortMap=u0,p1
  cfblk5 : DiscreteZeroPole  Poles=[0 0.5]  Gain=1
  cfblk6 : DiscreteStateSpace
  cfblk7 : MinMax
  cfblk8 : Math  Operator=magnitude^2
  cfblk9 : Sqrt  Operator=rSqrt  AlgorithmType=Newton-Raphson
  cfblk2 : Outport
  wires:
  cfblk11/1 -> cfblk10/1
  cfblk4/1 -> cfblk5/1
  cfblk1/1 -> cfblk11/1
  cfblk6/1 -> cfblk8/1
  cfblk13/1 -> cfblk3/1
  cfblk15/1 -> cfblk4/1
  cfblk14/1 -> cfblk6/1
  cfblk7/1 -> cfblk2/1
  cfblk8/1 -> cfblk4/2
  cfblk3/1 -> cfblk7/1
  cfblk5/1 -> cfblk9/1

== system sampleModel653/cfblk170/cfblk11 ==
  cfblk1 : Inport
  cfblk14 : Inport  Port=2
  cfblk15 : Inport  Port=3
  cfblk16 : Inport  Port=4
  cfblk10 : Gain  Gain=[865128015.575770]
  cfblk11 : ComplexToRealImag
  cfblk12 : simulink/Math Operations/MinMax Running Resettable  Function=min  vinit=0.0
  cfblk13 : Product
  cfblk18 : Delay  SampleTime=1
  cfblk19 : Delay  SampleTime=1
  cfblk3 : simulink/Discrete/Transfer Fcn Real Zero  ZeroZ=0.75  ICPrevInput=0.0  DoSatur=off
  cfblk4 : Delay  ShowEnablePort=on  SampleTime=1
      settings: InputPortMap=u0,e6
  cfblk5 : Delay  ShowEnablePort=on  SampleTime=1
      settings: InputPortMap=u0,e6
  cfblk6 : simulink/Discrete/Transfer Fcn Real Zero  ZeroZ=0.75  ICPrevInput=0.0  DoSatur=off
  cfblk7 : DiscreteIntegrator  ICPrevOutput=DiscIntNeverNeededParam  ICPrevScaledInput=DiscIntNeverNeededParam
  cfblk8 : simulink/Discrete/Transfer Fcn First Order  PoleZ=0.95  ICPrevOutput=0.0  DoSatur=off
  cfblk9 : Reshape
  cfblk2 : Outport
  cfblk17 : Outport  Port=2
  wires:
  cfblk6/1 -> cfblk9/1
  cfblk5/1 -> cfblk8/1
  cfblk3/1 -> cfblk5/1
  cfblk1/1 -> cfblk3/1
  cfblk12/1 -> cfblk11/1
  cfblk14/1 -> cfblk4/1
  cfblk11/1 -> cfblk7/1
  cfblk10/1 -> cfblk6/1
  cfblk11/2 -> cfblk13/1
  cfblk15/1 -> cfblk2/1
  cfblk4/1 -> cfblk12/2, cfblk17/1
  cfblk9/1 -> cfblk13/2
  cfblk8/1 -> cfblk4/2
  cfblk16/1 -> cfblk10/1
  cfblk7/1 -> cfblk18/1
  cfblk18/1 -> cfblk5/2
  cfblk13/1 -> cfblk19/1
  cfblk19/1 -> cfblk12/1

== system sampleModel653/cfblk170/cfblk12 ==
  cfblk1 : Inport
  cfblk3 : DiscreteIntegrator  ICPrevOutput=DiscIntNeverNeededParam  ICPrevScaledInput=DiscIntNeverNeededParam
  cfblk4 : simulink/Discrete/Transfer Fcn First Order  PoleZ=0.95  ICPrevOutput=0.0  DoSatur=off
  cfblk5 : Polyval  Coefs=[ +2.081618890e-019, -1.441693666e-014, +4.719686976e-010, -8.536869453e-006, +1.621573104e-001, -8.087801117e+001 ]
  cfblk6 : Gain  Gain=[-975229569.325468]
  cfblk7 : Math  Operator=conj
  cfblk2 : Outport
  cfblk8 : Outport  Port=2
  wires:
  cfblk6/1 -> cfblk7/1
  cfblk4/1 -> cfblk5/1
  cfblk7/1 -> cfblk3/1
  cfblk5/1 -> cfblk8/1, cfblk6/1
  cfblk1/1 -> cfblk4/1
  cfblk3/1 -> cfblk2/1

== system sampleModel653/cfblk171/cfblk6 ==
  cfblk1 : Inport
  cfblk15 : Inport  Port=2
  cfblk16 : Inport  Port=3
  cfblk10 : simulink/Math Operations/MinMax Running Resettable  Function=min  vinit=0.0
  cfblk11 : Product
  cfblk12 : Product
  cfblk13 : Product  Inputs=**
  cfblk14 : Constant  Value=[835907303.361022]  SampleTime=1
  cfblk17 : Delay  SampleTime=1
  cfblk3 : simulink/Discrete/Difference  ICPrevInput=0.0  OutMin=[]  OutMax=[]  OutDataTypeStr=Inherit: Inherit via back propagation  OutDataType=fixdt(1, 16)  OutScaling=2^-10  DoSatur=off
  cfblk4 : Delay  DelayLengthSource=Input port  SampleTime=1
      settings: InputPortMap=u0,p1
  cfblk5 : simulink/Discrete/Tapped Delay  vinit=0.0  samptime=-1  NumDelays=1  DelayOrder=Oldest  includeCurrent=off
  cfblk6 : simulink/Discrete/Transfer Fcn First Order  PoleZ=0.95  ICPrevOutput=0.0  DoSatur=off
  cfblk7 : Sqrt
  cfblk8 : ComplexToMagnitudeAngle
  cfblk9 : Product  Inputs=**
  cfblk2 : Outport
  wires:
  cfblk12/1 -> cfblk2/1
  cfblk6/1 -> cfblk12/1
  cfblk3/1 -> cfblk12/2
  cfblk11/1 -> cfblk5/1
  cfblk4/1 -> cfblk9/1
  cfblk14/1 -> cfblk8/1, cfblk4/2, cfblk10/2
  cfblk8/1 -> cfblk11/1
  cfblk5/1 -> cfblk3/1
  cfblk15/1 -> cfblk9/2
  cfblk8/2 -> cfblk6/1
  cfblk13/1 -> cfblk11/2
  cfblk16/1 -> cfblk13/1
  cfblk1/1 -> cfblk7/1
  cfblk7/1 -> cfblk10/1
  cfblk10/1 -> cfblk13/2
  cfblk9/1 -> cfblk17/1
  cfblk17/1 -> cfblk4/1

== system sampleModel653/cfblk171/cfblk7 ==
  cfblk1 : Inport
  cfblk6 : Inport  Port=2
  cfblk7 : Inport  Port=3
  cfblk3 : simulink/Discrete/Tapped Delay  vinit=0.0  samptime=-1  NumDelays=1  DelayOrder=Oldest  includeCurrent=off
  cfblk4 : Delay  DelayLengthSource=Input port  SampleTime=1
      settings: InputPortMap=u0,p1
  cfblk5 : UnaryMinus
  cfblk8 : Delay  SampleTime=1
  cfblk2 : Outport
  wires:
  cfblk3/1 -> cfblk5/1
  cfblk7/1 -> cfblk4/1
  cfblk1/1 -> cfblk2/1
  cfblk6/1 -> cfblk4/2
  cfblk5/1 -> cfblk8/1
  cfblk8/1 -> cfblk3/1

== system sampleModel653/cfblk172/cfblk5 ==
  cfblk1 : Inport
  cfblk9 : Inport  Port=2
  cfblk10 : Inport  Port=3
  cfblk11 : Inport  Port=4
  cfblk12 : Inport  Port=5
  cfblk14 : Delay  SampleTime=1
  cfblk3 : simulink/Discrete/Tapped Delay  vinit=0.0  samptime=-1  NumDelays=1  DelayOrder=Oldest  includeCurrent=off
  cfblk4 : MinMax
  cfblk5 : Trigonometry
  cfblk6 : Assignment  DiagnosticForDimensions=Warning  IndexOptions=Index vector (dialog)  Indices=1  OutputSizes=1
  cfblk7 : ComplexToRealImag
  cfblk8 : ComplexToMagnitudeAngle
  cfblk2 : Outport
  cfblk13 : Outport  Port=2
  wires:
  cfblk6/1 -> cfblk7/1
  cfblk8/1 -> cfblk3/1
  cfblk9/1 -> cfblk4/1
  cfblk10/1 -> cfblk6/1
  cfblk12/1 -> cfblk2/1
  cfblk1/1 -> cfblk5/1
  cfblk4/1 -> cfblk8/1
  cfblk7/2 -> cfblk13/1
  cfblk7/1 -> cfblk14/1
  cfblk14/1 -> cfblk6/2

== system sampleModel653/cfblk173/cfblk6 ==
  cfblk1 : Inport
  cfblk8 : Inport  Port=2
  cfblk3 : DiscreteFilter  SampleTime=1
  cfblk4 : Squeeze
  cfblk5 : Squeeze
  cfblk6 : ComplexToMagnitudeAngle
  cfblk7 : MinMax  Inputs=3
  cfblk2 : Outport
  cfblk9 : Outport  Port=2
  cfblk10 : Outport  Port=3
  wires:
  cfblk6/1 -> cfblk4/1
  cfblk8/1 -> cfblk2/1
  cfblk5/1 -> cfblk7/1, cfblk7/3
  cfblk7/1 -> cfblk10/1
  cfblk6/2 -> cfblk5/1
  cfblk4/1 -> cfblk3/1
  cfblk3/1 -> cfblk7/2
  cfblk1/1 -> cfblk6/1, cfblk9/1

== system sampleModel653/cfblk183/cfblk7 ==
  cfblk1 : Inport
  cfblk15 : Inport  Port=2
  cfblk16 : Inport  Port=3
  cfblk10 : Reshape
  cfblk11 : simulink/Math Operations/Slider Gain  gain=1  low=0  high=2
  cfblk12 : Constant  Value=[-867451952.968203]  SampleTime=1
  cfblk13 : Constant  Value=[815544775.062290]  SampleTime=1
  cfblk14 : Constant  Value=[-323296655.248306]  SampleTime=1
  cfblk18 : Delay
  cfblk3 : simulink/Discrete/Transfer Fcn Real Zero  ZeroZ=0.75  ICPrevInput=0.0  DoSatur=off
  cfblk4 : DiscreteZeroPole  Poles=[0 0.5]  Gain=1  SampleTime=-1
  cfblk5 : DiscreteFilter
  cfblk6 : Sum  Inputs=|++
  cfblk7 : Sqrt
  cfblk8 : ComplexToRealImag
  cfblk9 : simulink/Math Operations/Slider Gain  gain=1  low=0  high=2
  cfblk2 : Outport
  cfblk17 : Outport  Port=2
  wires:
  cfblk3/1 -> cfblk5/1
  cfblk9/1 -> cfblk11/1
  cfblk10/1 -> cfblk8/1
  cfblk6/1 -> cfblk4/1
  cfblk12/1 -> cfblk10/1
  cfblk7/1 -> cfblk9/1
  cfblk15/1 -> cfblk2/1
  cfblk11/1 -> cfblk17/1
  cfblk14/1 -> cfblk7/1
  cfblk5/1 -> cfblk6/1
  cfblk13/1 -> cfblk6/2
  cfblk4/1 -> cfblk18/1
  cfblk18/1 -> cfblk3/1

== system sampleModel653/cfblk184/cfblk10 ==
  cfblk1 : Inport
  cfblk11 : Inport  Port=2
  cfblk12 : Inport  Port=3
  cfblk13 : Inport  Port=4
  cfblk14 : Inport  Port=5
  cfblk10 : Constant  Value=[550729035.207121]  SampleTime=1
  cfblk3 : DiscreteStateSpace  SampleTime=-1
  cfblk4 : DiscreteTransferFcn
  cfblk5 : Delay  DelayLengthSource=Input port
      settings: InputPortMap=u0,p1
  cfblk6 : Sum  Inputs=|++
  cfblk7 : ComplexToMagnitudeAngle
  cfblk8 : Math  Operator=mod
  cfblk9 : Abs  SaturateOnIntegerOverflow=off
  cfblk2 : Outport
  cfblk15 : Outport  Port=2
  cfblk16 : Outport  Port=3
  wires:
  cfblk6/1 -> cfblk16/1
  cfblk4/1 -> cfblk8/1
  cfblk8/1 -> cfblk3/1
  cfblk10/1 -> cfblk8/2
  cfblk13/1 -> cfblk7/1
  cfblk11/1 -> cfblk9/1
  cfblk9/1 -> cfblk4/1
  cfblk3/1 -> cfblk2/1
  cfblk7/1 -> cfblk15/1
  cfblk12/1 -> cfblk5/1
  cfblk14/1 -> cfblk6/1
  cfblk5/1 -> cfblk6/2
  cfblk7/2 -> cfblk5/2

== system sampleModel653/cfblk184/cfblk11 ==
  cfblk1 : Inport
  cfblk11 : Inport  Port=2
  cfblk12 : Inport  Port=3
  cfblk13 : Inport  Port=4
  cfblk14 : Inport  Port=5
  cfblk15 : Inport  Port=6
  cfblk10 : Constant  Value=[-1640300.817515]  SampleTime=1
  cfblk16 : Delay
  cfblk3 : simulink/Discrete/Transfer Fcn Real Zero  ZeroZ=0.75  ICPrevInput=0.0  DoSatur=off
  cfblk4 : simulink/Discrete/Transfer Fcn Real Zero  ZeroZ=0.75  ICPrevInput=0.0  DoSatur=off
  cfblk5 : UnaryMinus
  cfblk6 : Squeeze
  cfblk7 : Sum  Inputs=+-
  cfblk8 : MinMax  Inputs=3
  cfblk9 : Bias  Bias=[960678397.132947]  SaturateOnIntegerOverflow=off
  cfblk2 : Outport
  wires:
  cfblk7/1 -> cfblk9/1
  cfblk5/1 -> cfblk7/1
  cfblk8/1 -> cfblk6/1
  cfblk14/1 -> cfblk2/1
  cfblk6/1 -> cfblk3/1
  cfblk12/1 -> cfblk4/1
  cfblk15/1 -> cfblk8/1
  cfblk13/1 -> cfblk5/1
  cfblk4/1 -> cfblk8/2
  cfblk10/1 -> cfblk8/3
  cfblk9/1 -> cfblk16/1
  cfblk16/1 -> cfblk7/2

== system sampleModel653/cfblk184/cfblk16 ==
  cfblk1 : Inport
  cfblk14 : Inport  Port=2
  cfblk15 : Inport  Port=3
  Action Port : ActionPort  ActionPortLabel=if(u1 >= 0)
  cfblk10 : simulink/Math Operations/Slider Gain  gain=1  low=0  high=2
  cfblk11 : Rounding
  cfblk12 : Trigonometry
  cfblk13 : Constant  Value=[-347633854.999822]  SampleTime=1
  cfblk3 : simulink/Discrete/Transfer Fcn Lead or Lag  PoleZ=0.95  ZeroZ=0.75  ICPrevOutput=0.0  ICPrevInput=0.0  DoSatur=off
  cfblk4 : Delay  DelayLengthSource=Input port
      settings: InputPortMap=u0,p1
  cfblk5 : Delay
  cfblk6 : Squeeze
  cfblk7 : Sqrt  Operator=rSqrt  AlgorithmType=Newton-Raphson
  cfblk8 : Trigonometry
  cfblk9 : Math  Operator=hypot
  cfblk2 : Outport
  cfblk16 : Outport  Port=2
  wires:
  cfblk14/1 -> cfblk6/1
  cfblk3/1 -> cfblk10/1
  cfblk1/1 -> cfblk11/1
  cfblk6/1 -> cfblk2/1
  cfblk8/1 -> cfblk4/1
  cfblk13/1 -> cfblk12/1
  cfblk4/1 -> cfblk9/1
  cfblk15/1 -> cfblk7/1
  cfblk10/1 -> cfblk4/2
  cfblk12/1 -> cfblk3/1
  cfblk7/1 -> cfblk5/1
  cfblk5/1 -> cfblk9/2
  cfblk11/1 -> cfblk8/1
  cfblk9/1 -> cfblk16/1

== system sampleModel653/cfblk184/cfblk17 ==
  cfblk1 : Inport
  cfblk8 : Inport  Port=2
  Action Port : ActionPort  ActionPortLabel=else
  cfblk10 : Delay
  cfblk3 : Product
  cfblk4 : ComplexToMagnitudeAngle
  cfblk5 : Product  Inputs=**
  cfblk6 : Reshape
  cfblk7 : Sum  Inputs=|++
  cfblk9 : Delay
  cfblk2 : Outport
  wires:
  cfblk3/1 -> cfblk4/1
  cfblk8/1 -> cfblk5/1
  cfblk6/1 -> cfblk5/2
  cfblk1/1 -> cfblk2/1
  cfblk4/1 -> cfblk7/1
  cfblk4/2 -> cfblk7/2
  cfblk7/1 -> cfblk6/1, cfblk9/1
  cfblk9/1 -> cfblk3/2
  cfblk5/1 -> cfblk10/1
  cfblk10/1 -> cfblk3/1

== system sampleModel653/cfblk184/cfblk9 ==
  cfblk1 : Inport
  cfblk10 : Inport  Port=2
  cfblk11 : Inport  Port=3
  cfblk12 : Inport  Port=4
  cfblk13 : Inport  Port=5
  cfblk14 : Inport  Port=6
  cfblk15 : Inport  Port=7
  cfblk17 : Delay
  cfblk3 : simulink/Discrete/Transfer Fcn Real Zero  ZeroZ=0.75  ICPrevInput=0.0  DoSatur=off
  cfblk4 : slpidlib/PID Controller  Controller=PID  Form=Parallel  TimeDomain=Discrete-time  UseExternalTs=off  SampleTime=-1  IntegratorMethod=Forward Euler  FilterMethod=Forward Euler  ControllerParametersSource=internal  P=1  I=1  UseKiTs=off  D=0  N=100  UseFilter=on  TunerSelectOption=Transfer Function Based (PID Tuner App)  InitialConditionSource=internal  InitialConditionForIntegrator=0  InitialConditionForFilter=0  DifferentiatorICPrevScaledInput=0  ExternalReset=none  TrackingMode=off  Kt=1  LimitOutput=off  SatLimitsSource=internal  UpperSaturationLimit=inf  LowerSaturationLimit=-inf  LinearizeAsGain=off  AntiWindupMode=none  Kb=1  LimitIntegrator=off  UpperIntegratorSaturationLimit=inf  LowerIntegratorSaturationLimit=-inf  POutMin=[]  POutMax=[]  IOutMin=[]  IOutMax=[]  DOutMin=[]  DOutMax=[]  NOutMin=[]  NOutMax=[]  SumOutMin=[]  SumOutMax=[]  SaturationOutMin=[]  SaturationOutMax=[]  PParamMin=[]  PParamMax=[]  IParamMin=[]  IParamMax=[]  DParamMin=[]  DParamMax=[]  NParamMin=[]  NParamMax=[]  KbParamMin=[]  KbParamMax=[]  KtParamMin=[]  KtParamMax=[]  KbOutMin=[]  KbOutMax=[]  KtOutMin=[]  KtOutMax=[]  IntegratorOutMin=[]  IntegratorOutMax=[]  FilterOutMin=[]  FilterOutMax=[]  SumI1OutMin=[]  SumI1OutMax=[]  SumI2OutMin=[]  SumI2OutMax=[]  SumI3OutMin=[]  SumI3OutMax=[]  SumI4OutMin=[]  SumI4OutMax=[]  SumDOutMin=[]  SumDOutMax=[]  DifferentiatorOutMin=[]  DifferentiatorOutMax=[]  FilterDiffOutCoefMin=[]  FilterDiffOutCoefMax=[]  ReciprocalOutMin=[]  ReciprocalOutMax=[]  SumDenOutMin=[]  SumDenOutMax=[]  SumNumOutMin=[]  SumNumOutMax=[]  DivideOutMin=[]  DivideOutMax=[]  UdiffTsProdOutMin=[]  UdiffTsProdOutMax=[]  NTsProdOutMin=[]  NTsProdOutMax=[]  UintegralTsProdOutMin=[]  UintegralTsProdOutMax=[]  UngainTsProdOutMin=[]  UngainTsProdOutMax=[]  ClampingZeroOutDataTypeStr=Inherit: Inherit via back propagation  ClampingZeroOutMin=[]  ClampingZeroOutMax=[]  FilterDenConstantOutDataTypeStr=Inherit: Inherit via back propagation  FilterDenConstantOutMin=[]  FilterDenConstantOutMax=[]  PCopyOutDataTypeStr=Inherit: Inherit via back propagation  PCopyOutMin=[]  PCopyOutMax=[]  NCopyOutDataTypeStr=Inherit: Inherit via back propagation  NCopyOutMin=[]  NCopyOutMax=[]  IntegratorContinuousStateAttributes=''  IntegratorStateMustResolveToSignalObject=off  IntegratorRTWStateStorageClass=Auto  FilterContinuousStateAttributes=''  FilterStateMustResolveToSignalObject=off  FilterRTWStateStorageClass=Auto  ParallelPVariant=InternalParameters  IdealPVariant=Disabled  IVariant=InternalParameters  DVariant=InternalParameters  IntegratorVariant=Discrete  SatVariant=Disabled  AWVariant=Passthrough  PCopyVariant=Disabled  TRVariant=Disabled  FdbkBlocksVariant=Forward  IdealPFdbkVariant=Disabled  SatFdbkVariant=Disabled  DerivativeFilterVariant=ForwardEulerFilter  NVariant=InternalParameters  NCopyVariant=Disabled  FilterICVariant=InternalICsFilter  IntegratorICVariant=InternalICs  ExternalResetVariant=Disabled  TRSumVariant=Passthrough  SumFdbkVariant=Disabled  SumVariant=Sum_PID  TsampFilterVariant=InternalTs  TsampNgainVariant=Passthrough  TsampIntegralVariant=Disabled_SignalSpec  ExternalSaturationOutDataTypeStr=Inherit: Same as second input
      settings: LibrarySourceBlock=simulink/Discrete/Discrete PID Controller
  cfblk5 : simulink/Discrete/Transfer Fcn Real Zero  ZeroZ=0.75  ICPrevInput=0.0  DoSatur=off
  cfblk6 : slpidlib/PID Controller (2DOF)  Controller=PID  Form=Parallel  TimeDomain=Discrete-time  UseExternalTs=off  SampleTime=-1  IntegratorMethod=Forward Euler  FilterMethod=Forward Euler  ControllerParametersSource=internal  P=1  I=1  UseKiTs=off  D=0  N=100  UseFilter=on  b=1  c=1  TunerSelectOption=Transfer Function Based (PID Tuner App)  InitialConditionSource=internal  InitialConditionForIntegrator=0  InitialConditionForFilter=0  DifferentiatorICPrevScaledInput=0  ExternalReset=none  TrackingMode=off  Kt=1  LimitOutput=off  SatLimitsSource=internal  UpperSaturationLimit=inf  LowerSaturationLimit=-inf  LinearizeAsGain=off  AntiWindupMode=none  Kb=1  LimitIntegrator=off  UpperIntegratorSaturationLimit=inf  LowerIntegratorSaturationLimit=-inf  POutMin=[]  POutMax=[]  IOutMin=[]  IOutMax=[]  DOutMin=[]  DOutMax=[]  NOutMin=[]  NOutMax=[]  bOutMin=[]  bOutMax=[]  cOutMin=[]  cOutMax=[]  SumOutMin=[]  SumOutMax=[]  SaturationOutMin=[]  SaturationOutMax=[]  PParamMin=[]  PParamMax=[]  IParamMin=[]  IParamMax=[]  DParamMin=[]  DParamMax=[]  NParamMin=[]  NParamMax=[]  bParamMin=[]  bParamMax=[]  cParamMin=[]  cParamMax=[]  KbParamMin=[]  KbParamMax=[]  KtParamMin=[]  KtParamMax=[]  KbOutMin=[]  KbOutMax=[]  KtOutMin=[]  KtOutMax=[]  IntegratorOutMin=[]  IntegratorOutMax=[]  FilterOutMin=[]  FilterOutMax=[]  SumI1OutMin=[]  SumI1OutMax=[]  SumI2OutMin=[]  SumI2OutMax=[]  SumI3OutMin=[]  SumI3OutMax=[]  SumI4OutMin=[]  SumI4OutMax=[]  SumDOutMin=[]  SumDOutMax=[]  Sum1OutMin=[]  Sum1OutMax=[]  Sum2OutMin=[]  Sum2OutMax=[]  Sum3OutMin=[]  Sum3OutMax=[]  DifferentiatorOutMin=[]  DifferentiatorOutMax=[]  FilterDiffOutCoefMin=[]  FilterDiffOutCoefMax=[]  ReciprocalOutMin=[]  ReciprocalOutMax=[]  SumDenOutMin=[]  SumDenOutMax=[]  SumNumOutMin=[]  SumNumOutMax=[]  DivideOutMin=[]  DivideOutMax=[]  UdiffTsProdOutMin=[]  UdiffTsProdOutMax=[]  NTsProdOutMin=[]  NTsProdOutMax=[]  UintegralTsProdOutMin=[]  UintegralTsProdOutMax=[]  UngainTsProdOutMin=[]  UngainTsProdOutMax=[]  ClampingZeroOutDataTypeStr=Inherit: Inherit via back propagation  ClampingZeroOutMin=[]  ClampingZeroOutMax=[]  FilterDenConstantOutDataTypeStr=Inherit: Inherit via back propagation  FilterDenConstantOutMin=[]  FilterDenConstantOutMax=[]  PCopyOutDataTypeStr=Inherit: Inherit via back propagation  PCopyOutMin=[]  PCopyOutMax=[]  NCopyOutDataTypeStr=Inherit: Inherit via back propagation  NCopyOutMin=[]  NCopyOutMax=[]  IntegratorContinuousStateAttributes=''  IntegratorStateMustResolveToSignalObject=off  IntegratorRTWStateStorageClass=Auto  FilterContinuousStateAttributes=''  FilterStateMustResolveToSignalObject=off  FilterRTWStateStorageClass=Auto  ParallelPVariant=InternalParameters  IdealPVariant=Disabled  IVariant=InternalParameters  DVariant=InternalParameters  bVariant=InternalParameters  cVariant=InternalParameters  IntegratorVariant=Discrete  SatVariant=Disabled  AWVariant=Passthrough  PCopyVariant=Disabled  TRVariant=Disabled  FdbkBlocksVariant=Forward  IdealPFdbkVariant=Disabled  SatFdbkVariant=Disabled  DerivativeFilterVariant=ForwardEulerFilter  NVariant=InternalParameters  NCopyVariant=Disabled  FilterICVariant=InternalICsFilter  IntegratorICVariant=InternalICs  ExternalResetVariant=Disabled  TRSumVariant=Passthrough  SumFdbkVariant=Disabled  SumVariant=Sum_PID  TsampFilterVariant=InternalTs  TsampNgainVariant=Passthrough  TsampIntegralVariant=Disabled_SignalSpec  ExternalSaturationOutDataTypeStr=Inherit: Same as second input
      settings: LibrarySourceBlock=simulink/Discrete/Discrete PID Controller (2DOF)
  cfblk7 : DiscreteTransferFcn
  cfblk8 : simulink/Discrete/Transfer Fcn First Order  PoleZ=0.95  ICPrevOutput=0.0  DoSatur=off
  cfblk9 : Bias  Bias=[563309978.821048]  SaturateOnIntegerOverflow=off
  cfblk2 : Outport
  cfblk16 : Outport  Port=2
  wires:
  cfblk5/1 -> cfblk7/1
  cfblk12/1 -> cfblk5/1
  cfblk4/1 -> cfblk8/1
  cfblk10/1 -> cfblk16/1
  cfblk7/1 -> cfblk4/1
  cfblk15/1 -> cfblk6/1
  cfblk1/1 -> cfblk9/1
  cfblk3/1 -> cfblk6/2
  cfblk11/1 -> cfblk2/1
  cfblk6/1 -> cfblk17/1
  cfblk17/1 -> cfblk3/1
